simulink model "Lab2_single_loop_controller_student"  (R2025a)
settings: Solver=ode45  StartTime=0.0  StopTime=10  FixedStep=0.001  MaxStep=0.01  RelTol=1e-3
values from neighbouring files (symbols this model uses):
  g = 9.81    [Lab2_params_student.m]
  J = 0.000058559    (= 5.8559e-05)    [Lab2_params_student.m]    (also in part1.m = 1.307e-05)
  Kd = 0.46716    [Lab2_params_student.m]
  ke = 0.0528    [Lab2_params_student.m]    (also in part1.m = 0.0473)
  Ki = 0.6840    (= 0.684)    [Lab2_params_student.m]
  Kp = 1.1305    [Lab2_params_student.m]
  kt = 0.0506    [Lab2_params_student.m]    (also in part1.m = 0.0473)
  L = 0.1    [Lab2_params_student.m]
  Lm = 0.0028445    [Lab2_params_student.m]    (also in part1.m = 0.003384)
  mp = 0.05    [Lab2_params_student.m]
  R = 3.18    [Lab2_params_student.m]    (also in part1.m = 5.52186)
  s = tf('s')    [part1.m]
undefined symbols (not defined in the file or in its folder): X, Y, Z
libraries: sm_lib x28, nesl_utility x8, slpidlib x1
(part 1 of 2)
settings Model: Creator=User  LastModifiedBy=eak_s
settings RTWCC: GPUComputeCapability=3.5

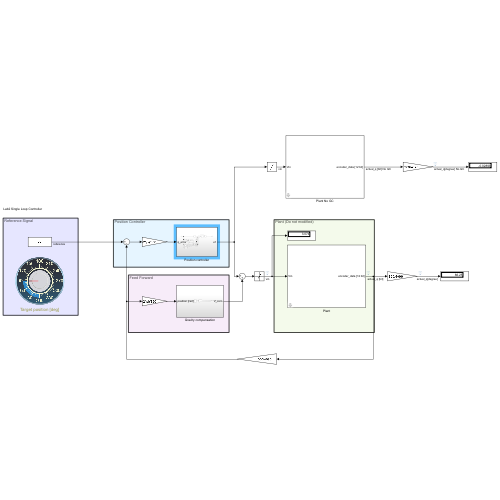
[thumbnail: Simulink's stored preview of the top-level diagram]
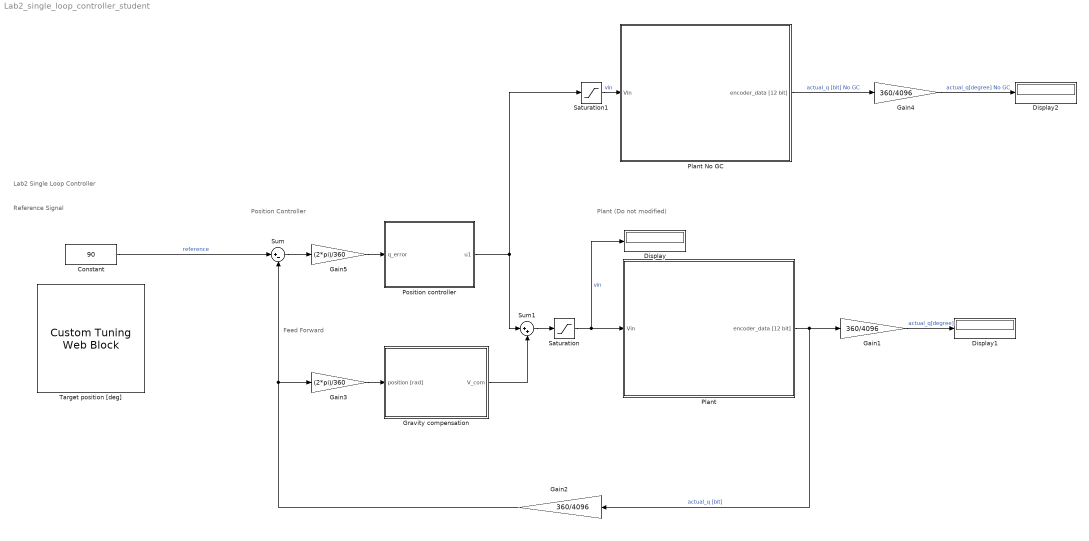
== system Lab2_single_loop_controller_student ==
  note: Lab2 Single Loop Controller
  note: Plant (Do not modified)
  note: Feed Forward
  note: Position Controller
  note: Reference Signal
  Constant : Constant  Value=90  SampleTime=-1
  Display : Display
  Display1 : Display
  Display2 : Display
  Gain1 : Gain  Gain=360/4096
  Gain2 : Gain  Gain=360/4096
  Gain3 : Gain  Gain=(2*pi)/360
  Gain4 : Gain  Gain=360/4096
  Gain5 : Gain  Gain=(2*pi)/360
  Gravity compensation : Subsystem
  Plant : Subsystem  mask{init_q=0}
      mask prompts: init_q "Initial angle of pendulum [deg]"
  Plant No GC : Subsystem  mask{init_q=0}
      mask prompts: init_q "Initial angle of pendulum [deg]"
  Position controller : Subsystem
  Saturation : Saturate  UpperLimit=12  LowerLimit=-12
  Saturation1 : Saturate  UpperLimit=12  LowerLimit=-12
  Sum : Sum  Inputs=|+-
  Sum1 : Sum  Inputs=|++
  Target position [deg] : CustomTuningWebBlock  LabelPosition=Hide  ShowInitialText=on  Configuration="{\"components\":[{\"name\":\"CircularScaleComponent\",\"settings\":{\"bounds\":{\"max\":360,\"min\":0,\"tickInterval\":30},\"direction\":\"cw\",\"flipLimits\":0,\"innerRadius\":0.6636618227670849,\"internalTickHeightScaleFactor\":1,\"labelColor\":[255,255,200],\"labelFont\":{\"font\":\"Arial\",\"fontSize\":12},\"labelRadius\":0.79,\"labelTransparency\":1,\"minorTickHeightScaleFactor\":0.2,\"needleImage\":{\"size\":[150,150],\"src\":\"data:image\\/svg+xml;base64,PD94bWwgdmVyc2lvbj0iMS4wIiBlbmNvZGluZz0idXRmLTgiPz4NCjwhLS0gR2VuZXJhdG9yOiBBZG9iZSBJbGx1c3RyYXRvciAyNS4yLjMsIFNWRyBFeHBvcnQgUGx1Zy1JbiAuIFNWRyBWZXJzaW9uOiA2LjAwIEJ1aWxkIDApICAtLT4NCjxzdmcgdmVyc2lvbj0iMS4xIiBpZD0iTGF5ZXJfMSIgeG1sbnM9Imh0dHA6Ly93d3cudzMub3JnLzIwMDAvc3ZnIiB4bWxuczp4bGluaz0iaHR0cDovL3d3dy53My5vcmcvMTk5OS94bGluayIgeD0iMHB4IiB5PSIwcHgiDQoJIHZpZXdCb3g9IjAgMCAxNTIgMTUyIiBzdHlsZT0iZW5hYmxl ...(+37472 chars)\"},\"needleOffset\":[0,0],\"needleOrientation\":-45,\"needleRotation\":90,\"needleSize\":{\"height\":0.44,\"width\":0.44},\"outerRadius\":0.5053386200069245,\"position\":[0,0,1,1],\"referencePoint\":\"auto\",\"scaleAngle\":360,\"scaleAngleOffset\":90,\"scaleColors\":[],\"scaleColorsSize\":0.2,\"scaleDirection\":\"CW\",\"scalePosition\":[0,0,1,1],\"showLabels\":1,\"showMinorTicks\":1,\"showSpanLine\":true,\"showTicks\":1,\"tickColor\":[252,252,197],\"tickTransparency\":1,\"valueBarColor\":[0,114,189],\"valueBarPosition\":[0,0,1,1],\"valueBarSize\":0.2,\"valueBarTransparency\":1}},{\"name\":\"BackgroundImageComponent\",\"settings\":{\"image\":{\"size\":[385,373],\"src\":\"data:image\\/svg+xml;base64,PD94bWwgdmVyc2lvbj0iMS4wIiBlbmNvZGluZz0idXRmLTgiPz4NCjwhLS0gR2VuZXJhdG9yOiBBZG9iZSBJbGx1c3RyYXRvciAyNS4wLjAsIFNWRyBFeHBvcnQgUGx1Zy1JbiAuIFNWRyBWZXJzaW9uOiA2LjAwIEJ1aWxkIDApICAtLT4NCjxzdmcgdmVyc2lvbj0iMS4xIg0KCSBpZD0iTGF5ZXJfMl8xXyIgeG1sbnM6Y2M9Imh0dHA6Ly9jcmVhdGl2ZWNvbW1vbnMub3JnL25zIyIgeG1sbnM6ZGM9Imh0dHA6Ly9wdXJsLm9yZy9kYy9lbGVtZW50cy8xLjEvIiB4bWxuczppbmtzY2FwZT0iaHR0cDovL3d3dy5pbmtzY2FwZS5vcmcv ...(+4184 chars)\",\"srcOrientation\":\"horizontal\"},\"position\":[0,0,1,1],\"scaleMode\":\"0\"}},{\"name\":\"ForegroundImageComponent\",\"settings\":{\"image\":{\"size\":[0,0],\"src\":\"default\",\"srcOrientation\":[]},\"isForeground\":1,\"position\":[0,0,1,1],\"scaleMode\":\"0\"}}],\"derived\":{\"blockParameters\":{\"ForegroundColor\":[0.9882352941176471,0.9882352941176471,0.7725490196078432],\"Limits\":{\"Max\":360,\"Min\":0,\"Ticks\":30},\"ScaleColors\":[],\"ScaleDirection\":\"Clockwise\",\"ScaleMax\":360,\"ScaleMin\":0,\"TickInterval\":30,\"fixedAspectRatio\":\"off\"}},\"settings\":{\"BindingType\":\"param\",\"aspectRatio\":1,\"backgroundColor\":[0,0,0,\"1\"],\"backgroundOffset\":1,\"backgroundOpacity\":1,\"direction\":\"cw\",\"fixedAspectRatio\":\"off\",\"flipLimits\":0,\"foregroundColor\":[252,252,196],\"orientation\":\"horizontal\",\"showBackgroundColor\":false,\"value\":0,\"version\":\"R2023a\"},\"type\":\"CircularGauge\"}"
  wires:
  Saturation/1 -> Display/1, Plant/1(Vin)  "vin"
  Constant/1 -> Sum/1  "reference"
  Plant/1(encoder_data [12 bit]) -> Gain1/1, Gain2/1  "actual_q [bit]"
  Sum/1 -> Gain5/1
  Sum1/1 -> Saturation/1
  Position controller/1(u1) -> Saturation1/1, Sum1/1
  Gain1/1 -> Display1/1  "actual_q[degree]"
  Gravity compensation/1(V_com) -> Sum1/2
  Gain2/1 -> Gain3/1, Sum/2
  Gain3/1 -> Gravity compensation/1(position [rad])
  Saturation1/1 -> Plant No GC/1(Vin)  "vin"
  Plant No GC/1(encoder_data [12 bit]) -> Gain4/1  "actual_q [bit] No GC"
  Gain4/1 -> Display2/1  "actual_q[degree] No GC"
  Gain5/1 -> Position controller/1(q_error)

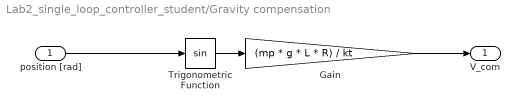
== system Lab2_single_loop_controller_student/Gravity compensation ==
  position [rad] : Inport
  Gain : Gain  Gain=(mp * g * L * R) / kt
  Trigonometric Function : Trigonometry
  V_com : Outport
  wires:
  Trigonometric Function/1 -> Gain/1
  Gain/1 -> V_com/1
  position [rad]/1 -> Trigonometric Function/1

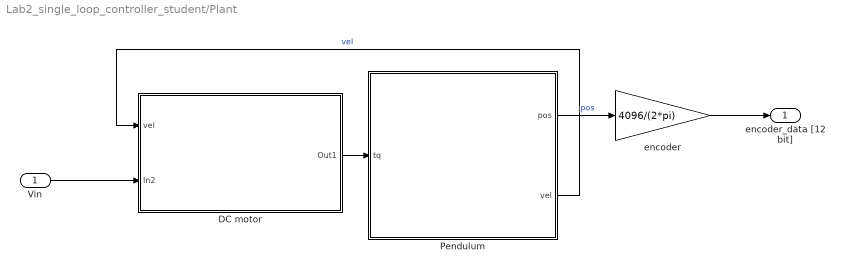
== system Lab2_single_loop_controller_student/Plant ==
  Vin : Inport
  DC motor : Subsystem
  Pendulum : Subsystem
      mask Display: image('simple_pendulum_brick.png'); % Use "Edit Image" on toolstrip to change.
  encoder : Gain  Gain=4096/(2*pi)
  encoder_data [12 bit] : Outport
  wires:
  Pendulum/1(pos) -> encoder/1  "pos"
  encoder/1 -> encoder_data [12 bit]/1
  Pendulum/2(vel) -> DC motor/1(vel)  "vel"
  Vin/1 -> DC motor/2(In2)
  DC motor/1(Out1) -> Pendulum/1(tq)

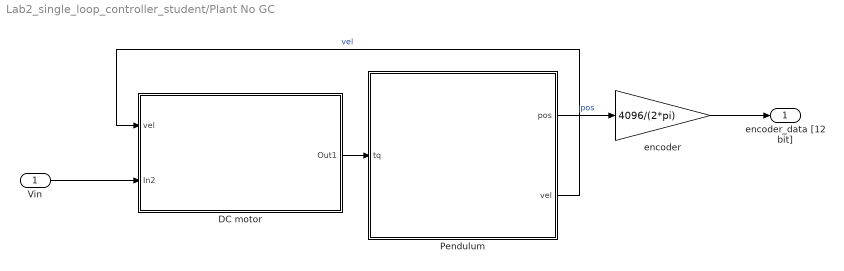
== system Lab2_single_loop_controller_student/Plant No GC ==
  Vin : Inport
  DC motor : Subsystem
  Pendulum : Subsystem
      mask Display: image('simple_pendulum_brick.png'); % Use "Edit Image" on toolstrip to change.
  encoder : Gain  Gain=4096/(2*pi)
  encoder_data [12 bit] : Outport
  wires:
  Pendulum/1(pos) -> encoder/1  "pos"
  encoder/1 -> encoder_data [12 bit]/1
  Pendulum/2(vel) -> DC motor/1(vel)  "vel"
  Vin/1 -> DC motor/2(In2)
  DC motor/1(Out1) -> Pendulum/1(tq)
